simulink library "algebraic_method"  (R2021b)
settings: Solver=VariableStepAuto  StartTime=0.0  StopTime=10.0  RelTol=1e-3
settings Model: Creator=white  LastModifiedBy=white

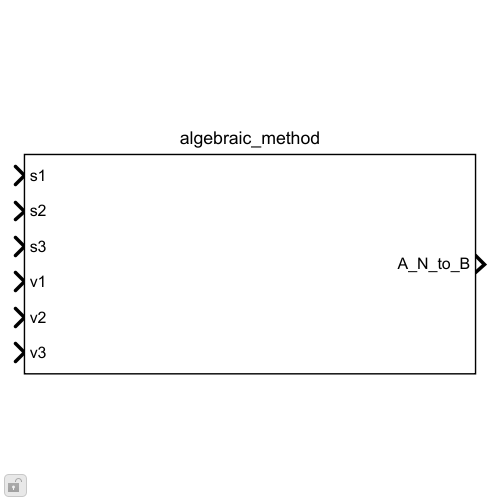
[thumbnail: Simulink's stored preview of the top-level diagram]
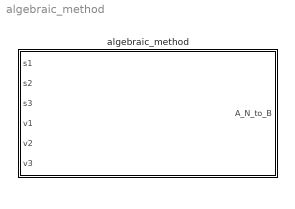
== system algebraic_method ==
  algebraic_method : Subsystem

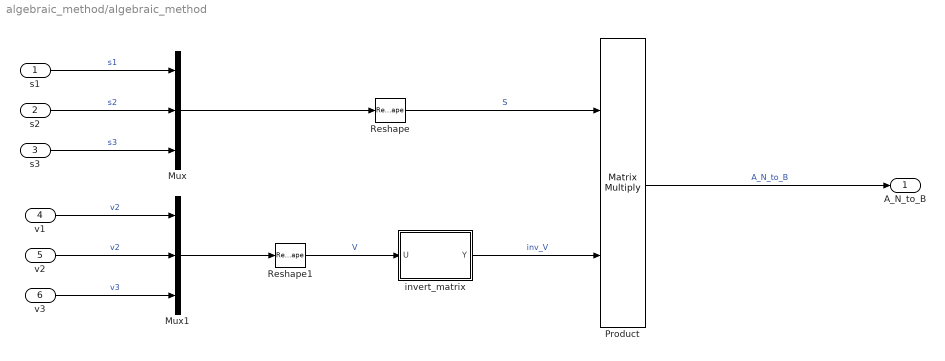
== system algebraic_method/algebraic_method ==
  s1 : Inport
  s2 : Inport  Port=2
  s3 : Inport  Port=3
  v1 : Inport  Port=4
  v2 : Inport  Port=5
  v3 : Inport  Port=6
  Mux : Mux  Inputs=3
  Mux1 : Mux  Inputs=3
  Product : Product  Multiplication=Matrix(*)
  Reshape : Reshape  OutputDimensionality=Customize  OutputDimensions=[3,3]
  Reshape1 : Reshape  OutputDimensionality=Customize  OutputDimensions=[3,3]
  invert_matrix : MATLAB Function  TreatAsAtomicUnit=on
  A_N_to_B : Outport
  wires:
  Product/1 -> A_N_to_B/1  "A_N_to_B"
  invert_matrix/1(Y) -> Product/2  "inv_V"
  Mux1/1 -> Reshape1/1
  Mux/1 -> Reshape/1
  s3/1 -> Mux/3  "s3"
  s2/1 -> Mux/2  "s2"
  s1/1 -> Mux/1  "s1"
  v1/1 -> Mux1/1  "v2"
  v2/1 -> Mux1/2  "v2"
  v3/1 -> Mux1/3  "v3"
  Reshape/1 -> Product/1  "S"
  Reshape1/1 -> invert_matrix/1(U)  "V"

== matlab function algebraic_method/invert_matrix ==
  data: U input; Y output
function Y = invert(U)

Y = inv(U);
